simulink model "SimFuzzyPID"  (R2017a)
settings: Solver=FixedStepDiscrete  StartTime=0.0  StopTime=12  RelTol=1e-3  EnableMultiTasking=on
PreLoadFcn:
  | Ts = 0.1;
  | Plant = c2d(zpk([],[-1 -3 -5],1),Ts);
  | C0 = pid(1,1,1,'Ts',Ts,'IF','B','DF','B'); % define PID structure
  | C = pidtune(Plant,C0); % design PID
  | [Kp Ki Kd] = piddata(C); % obtain PID gains
  | FIS = newfis('FIS','sugeno');
  | FIS = addvar(FIS,'input','E',[-10 10]);
  | FIS = addmf(FIS,'input',1,'Negative','gaussmf',[7 -10]);
  | FIS = addmf(FIS,'input',1,'Positive','gaussmf',[7 10]);
  | FIS = addvar(FIS,'input','CE',[-10 10]);
  | FIS = addmf(FIS,'input',2,'Negative','gaussmf',[7 -10]);
  | FIS = addmf(FIS,'input',2,'Positive','gaussmf',[7 10]);
  | FIS = addvar(FIS,'output','u',[-20 20]);
  | FIS = addmf(FIS,'output',1,'Min','constant',-20);
  | FIS = addmf(FIS,'output',1,'Zero','constant',0);
  | FIS = addmf(FIS,'output',1,'Max','constant',20);
  | ruleList = [1 1 1 1 1;...   % Rule 1
  |             1 2 2 1 1;...   % Rule 2
  |             2 1 2 1 1;...   % Rule 3
  |             2 2 3 1 1];     % Rule 4
  | FIS = addrule(FIS,ruleList);GE = 10;
  | GCE = GE*(Kp-sqrt(Kp^2-4*Ki*Kd))/2/Ki;
  | GCU = Ki/GE;
  | GU = Kd/GCE;
  | Step = 1; % use 21 break points for both E and CE inputs
  | E = -10:Step:10;
  | CE = -10:Step:10;
  | N = length(E);
  | LookUpTableData = zeros(N);
  | for i=1:N
  |    for j=1:N
  |       % compute output u for each combination of break points
  |       LookUpTableData(i,j) = evalfis([E(i) CE(j)],FIS);
  |    end
  | end
undefined symbols (not defined in the file or in its folder): DiscIntNeverNeededParam, Kd, Ki, Kp
libraries: simulink x2, cstblocks x2, fuzblock x1
settings Model: FPTRunName=Active  Creator=The MathWorks, Inc.  LastModifiedBy=Alfian Fadli P
settings DataIOCC: LimitDataPoints=on  SaveFormat=Array
settings OptimizationCC: ExpressionDepthLimit=2147483647  LifeSpan=inf
settings DebuggingCC: UnderspecifiedInitializationDetection=Classic  MergeDetectMultiDrivingBlocksExec=none  SolverPrmCheckMsg=warning  FcnCallInpInsideContextMsg=warning  StateNameClashWarn=warning  SFUnexpectedBacktrackingDiag=warning  SFNoUnconditionalDefaultTransitionDiag=warning  SFExecutionAtInitializationDiag=none
settings HardwareCC: ProdBitPerPointer=32  ProdBitPerSizeT=32  ProdBitPerPtrDiffT=32  ProdLargestAtomicFloat=None  ProdIntDivRoundTo=Undefined  ProdEndianess=Unspecified  ProdWordSize=32  ProdHWDeviceType=32-bit Generic
settings ModelReferenceCC: PropagateSignalLabelsOutOfModel=off
settings GRTTargetCC: TargetLangStandard=C89/C90 (ANSI)  GeneratePreprocessorConditionals=Disable all  CombineOutputUpdateFcns=off  GRTInterface=on
settings ConfigComp: CovMetricSettings=dw  CovHtmlReporting=on  CovSaveCumulativeToWorkspaceVar=on  CovSaveSingleToWorkspaceVar=on  CovExternalEMLEnable=off

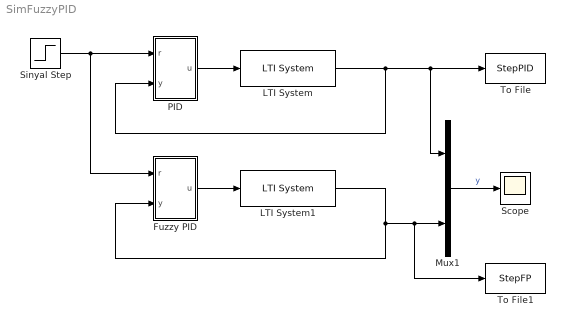
== system SimFuzzyPID ==
  Fuzzy PID : Subsystem
  LTI System : cstblocks/LTI System  sys=Plant  IC=[]
  LTI System1 : cstblocks/LTI System  sys=Plant  IC=[]
  Mux1 : Mux  Inputs=2
  PID : Subsystem
  Scope : Scope
  Sinyal Step : Step  SampleTime=0
  To File : ToFile  Filename=StepPID  MatrixName=StepPID
  To File1 : ToFile  Filename=StepFP  MatrixName=StepFP
  wires:
  LTI System/1 -> PID/2(y), To File/1, Mux1/1
  PID/1(u) -> LTI System/1
  Sinyal Step/1 -> Fuzzy PID/1(r), PID/1(r)
  LTI System1/1 -> Fuzzy PID/2(y), To File1/1, Mux1/2
  Fuzzy PID/1(u) -> LTI System1/1
  Mux1/1 -> Scope/1  "y"

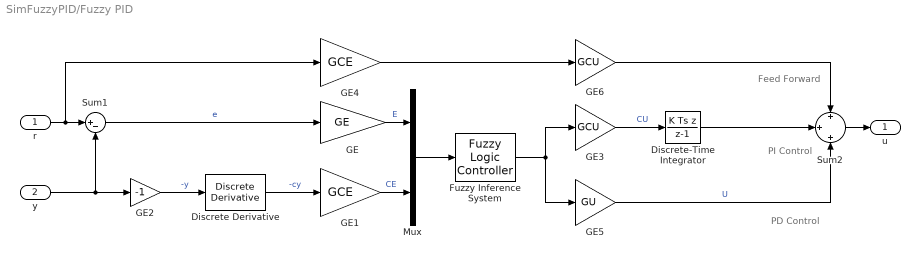
== system SimFuzzyPID/Fuzzy PID ==
  note: PD Control
  note: PI Control
  note: Feed Forward
  r : Inport
  y : Inport  Port=2
  Discrete Derivative : simulink/Discrete/Discrete Derivative  gainval=1  ICPrevScaledInput=0.0  InputProcessing=Inherited  OutMin=[]  OutMax=[]  OutDataType=fixdt(1, 16)  OutScaling=2^-10  DoSatur=off
  Discrete-Time Integrator : DiscreteIntegrator  IntegratorMethod=Integration: Backward Euler  SampleTime=Ts  ICPrevOutput=DiscIntNeverNeededParam  ICPrevScaledInput=DiscIntNeverNeededParam
  Fuzzy Inference System : fuzblock/Fuzzy Logic  Controller  fis=FIS
  GE : Gain  Gain=GE
  GE1 : Gain  Gain=GCE
  GE2 : Gain  Gain=-1
  GE3 : Gain  Gain=GCU
  GE4 : Gain  Gain=GCE
  GE5 : Gain  Gain=GU
  GE6 : Gain  Gain=GCU
  Mux : Mux  Inputs=2
  Sum1 : Sum  Inputs=|+-
  Sum2 : Sum  Inputs=+|+|+
  u : Outport
  wires:
  Sum1/1 -> GE/1  "e"
  Mux/1 -> Fuzzy Inference System/1
  GE/1 -> Mux/1  "E"
  GE1/1 -> Mux/2  "CE"
  Fuzzy Inference System/1 -> GE3/1, GE5/1
  GE3/1 -> Discrete-Time Integrator/1  "CU"
  GE5/1 -> Sum2/3  "U"
  GE2/1 -> Discrete Derivative/1  "-y"
  Discrete Derivative/1 -> GE1/1  "-cy"
  r/1 -> Sum1/1, GE4/1
  y/1 -> Sum1/2, GE2/1
  Sum2/1 -> u/1
  GE4/1 -> GE6/1
  Discrete-Time Integrator/1 -> Sum2/2
  GE6/1 -> Sum2/1

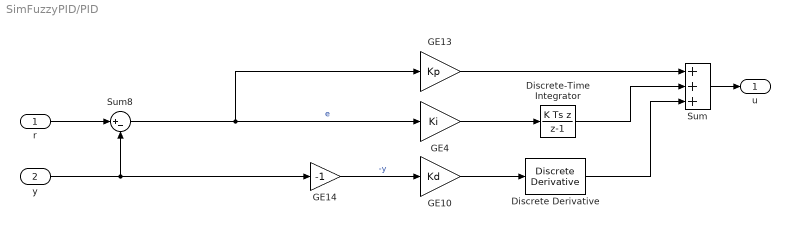
== system SimFuzzyPID/PID ==
  r : Inport
  y : Inport  Port=2
  Discrete Derivative : simulink/Discrete/Discrete Derivative  gainval=1  ICPrevScaledInput=0.0  InputProcessing=Inherited  OutMin=[]  OutMax=[]  OutDataType=fixdt(1, 16)  OutScaling=2^-10  DoSatur=off
  Discrete-Time Integrator : DiscreteIntegrator  IntegratorMethod=Integration: Backward Euler  gainval=1  SampleTime=Ts  ICPrevOutput=DiscIntNeverNeededParam  ICPrevScaledInput=DiscIntNeverNeededParam
  GE10 : Gain  Gain=Kd
  GE13 : Gain  Gain=Kp
  GE14 : Gain  Gain=-1
  GE4 : Gain  Gain=Ki
  Sum : Sum  Inputs=+++
  Sum8 : Sum  Inputs=|+-
  u : Outport
  wires:
  GE13/1 -> Sum/1
  Sum8/1 -> GE4/1, GE13/1  "e"
  Discrete-Time Integrator/1 -> Sum/2
  GE4/1 -> Discrete-Time Integrator/1
  GE10/1 -> Discrete Derivative/1
  Discrete Derivative/1 -> Sum/3
  GE14/1 -> GE10/1  "-y"
  r/1 -> Sum8/1
  y/1 -> Sum8/2, GE14/1
  Sum/1 -> u/1
